simulink model "ssc_auto_ev_20b"  (R2020b)
settings: Solver=VariableStepAuto  StartTime=0.0  StopTime=200  RelTol=1e-3  AbsTol=1e-3
PreLoadFcn:
  | % Simulation parameters
  | dt = 0.01;
  | 
  | % Battery cell parameters
  | ssc_lithium_cell_1RC_ini
  | Nseries = 100;
  | Nparallel = 10;
  | 
  | % Motor parameters
  | max_torque = 220;
  | max_power = 80e3;
  | 
  | % Vehicle parameters
  | vehicle_mass = 4000;
  | wheel_radius = 0.35;
  | area = 5;
  | drag_coefficient = 0.25;
  | air_density = 1.225;
  | gravity = 9.81;
  | rolling_res_ratio = 0.015;
  | 
  | % Differential drive parameters
  | gear_ratio = 12;
  | 
  | % Simplified braking system parameters
  | force_max_pedal = 500;
  | braking_torque_to_pedal_force_ratio = -16;
  | 
  | % Vehicle controller parameters
  | hill_hold_max_speed = 0.5;
  | 
  | % Water properties for cooling circuit
  | load WaterProperties
  | 
  | % Input signals for Signal Editor block
  | load ssc_auto_ev_Inputs
values from neighbouring files (symbols this model uses):
  C1_LUT = [1913.6 4625.7 23306 10736 18036 12251 9022.9 12447 18872 40764 18721 33630 ... (21 elements, 7x3)]    [ssc_auto_ev_param.mat]
  Capacity_LUT = [28.0081 27.625 27.6392]    [ssc_auto_ev_param.mat]
  cell_Cp_heat = 810.5328    [ssc_auto_ev_param.mat]
  cell_mass = 1    [ssc_auto_ev_param.mat]
  Em_LUT = [3.4966 3.5519 3.6183 3.7066 3.9131 4.0748 4.1923 3.5057 3.566 3.6337 3.7127 3.9259 ... (21 elements, 7x3)]    [ssc_auto_ev_param.mat]
  Qe_init = 15.6845    [ssc_auto_ev_param.mat]
  R0_LUT = [0.0117 0.011 0.0114 0.0107 0.0107 0.0113 0.0116 0.0085 0.0085 0.0087 0.0082 0.0083 ... (21 elements, 7x3)]    [ssc_auto_ev_param.mat]
  R1_LUT = [0.0109 0.0069 0.0047 0.0034 0.0033 0.0033 0.0028 0.0029 0.0024 0.0026 0.0016 0.0023 ... (21 elements, 7x3)]    [ssc_auto_ev_param.mat]
  SOC_LUT = [0 0.1 0.25 0.5 0.75 0.9 1]    [ssc_auto_ev_param.mat]
  T_init = 293.15    [ssc_auto_ev_param.mat]
  Temperature_LUT = [278.15 293.15 313.15]    [ssc_auto_ev_param.mat]
undefined symbols (not defined in the file or in its folder): DiscIntNeverNeededParam, K, Lambda, tau, x0
libraries: fl_lib x656, nesl_utility x86, simulink x21, LiBatteryElements_lib x16, SignalEditorBlockLib x4, simulink_extras x4
(part 7 of 13)

== system ssc_auto_ev_20b/Step 4: Deployment Model/Vehicle and drive @100Hz ==
  Test data : Inport
  iRef : Inport  Port=2
  voltage : Inport  Port=3
  heat flow : Inport  Port=4
  heat flow1 : Inport  Port=5
  ERef2 : fl_lib/Electrical/Electrical Elements/Electrical Reference
      settings: SourceProductBaseCode=PW,SS,VE
  Motor Drive : Subsystem  Tag=PublishSubsystem  VariantControl=Variant1
  Port 1 Interface1 : Subsystem  mask(Network Coupler (Thermal Mass) Port 1 Interface){thermalMass=10*447, samplingType=physmod:simscape:couplers:SimscapeNetworkCouplersLib:VariableStepAtPorts1And2_PV, h1=dt, h2=dt*5, predictionDiscreteToContinuous=off, smoothingContinuousToDiscrete=off, predictionSlowToFast=off, smoothingFastToSlow=off, nSmooth=1, tsSmoothing=0.01, thermalConductanceNetwork=1, hRecommended=0.001, T0=T_init}
      mask prompts: thermalMass "physmod:simscape:couplers:SimscapeNetworkCouplersLib:ThermalMassJK_MP"; samplingType "physmod:simscape:couplers:SimscapeNetworkCouplersLib:SamplingType_MP"; h1 "physmod:simscape:couplers:SimscapeNetworkCouplersLib:Port1NetworkDiscreteSampleTimes_MP"; h2 "physmod:simscape:couplers:SimscapeNetworkCouplersLib:Port2NetworkDiscreteSampleTimes_MP"; predictionDiscreteToContinuous "physmod:simscape:couplers:SimscapeNetworkCouplersLib:UsePredictionWhenConnectingFixedStepToVariableStep_MP"; smoothingContinuousToDiscrete "physmod:simscape:couplers:SimscapeNetworkCouplersLib:UseSmoothingWhenConnectingVariableStepToFixedStep_MP"; predictionSlowToFast "physmod:simscape:couplers:SimscapeNetworkCouplersLib:UsePredictionWhenConnectingSlowToFastSampleTimes_MP"; smoothingFastToSlow "physmod:simscape:couplers:SimscapeNetworkCouplersLib:UseSmoothingWhenConnectingFastToSlowSampleTimes_MP"; nSmooth "physmod:simscape:couplers:SimscapeNetworkCouplersLib:NumberOfSamplesOverWhichToSmooth_MP"; tsSmoothing "physmod:simscape:couplers:SimscapeNetworkCouplersLib:SmoothingTimeConstants_MP"; thermalConductanceNetwork "physmod:simscape:couplers:SimscapeNetworkCouplersLib:ApproximateConnectedNetworkThermalConductanceWK_MP"; hRecommended "physmod:simscape:couplers:SimscapeNetworkCouplersLib:RecommendedMaxDiscreteSampleTimes_MP"; T0 "physmod:simscape:couplers:SimscapeNetworkCouplersLib:InitialTemperatureK_MP"
      mask help: physmod:simscape:couplers:SimscapeNetworkCouplersLib:NetworkCouplerThermalMassPort1Interface_MD
      mask init: same as ssc_auto_ev_20b/Step 3: Ungroup and Redraw/Port 1 Interface1
      settings: PortSchema="{\"entries\":[{\"content\":{\"sides\":[{\"content\":{\"connectorIds\":[\"LConn1\"]},\"type\":\"ConnectorPlacement.EquallySpacedRectSide\",\"uuid\":\"a6d4a9fd-b5aa-40dc-ab7e-2b646b9b57bc\"},{\"content\":{\"connectorIds\":[\"Out1\",\"In1\"],\"side\":\"RIGHT\"},\"type\":\"ConnectorPlacement.EquallySpacedRectSide\",\"uuid\":\"31bb6273-5b9b-48d0-a1a2-6fbacb979b97\"},{\"content\":{\"connectorIds\":[],\"side\":\"TOP\"},\"type\":\"ConnectorPlacement.EquallySpacedRectSide\",\"uuid\":\"0f7afab2-4481-486c-9ad0-2b42c5b091a4\"}]},\"type\":\"ConnectorPlacement.EquallySpacedConnector\",\"uuid\":\"a98e47aa-cbfd-441a-b14c-c9ea515c056e\"}],\"packageUris\":[\"http://schema.mathworks.com/mf0/Connector/R2020b\"],\"version\":\"1.0\"}"
      mask Help: web([docroot '/physmod/simscape/ref/networkcouplerthermalmass.html'])
      mask TypeOptions samplingType: physmod:simscape:couplers:SimscapeNetworkCouplersLib:VariableStepAtPorts1And2_PV | physmod:simscape:couplers:SimscapeNetworkCouplersLib:VariableStepAtPort1AndFixedStepAtPort2_PV | physmod:simscape:couplers:SimscapeNetworkCouplersLib:FixedStepBothPortsWithCommonSampleTime_PV | physmod:simscape:couplers:SimscapeNetworkCouplersLib:FixedStepBothPortsWithFasterSamplingAtPort1_PV
      mask Callback samplingType: foundation.internal.couplers.thermal.parameterVisibilitiesThermalMass(gcb)
      mask Callback predictionDiscreteToContinuous: foundation.internal.couplers.thermal.parameterVisibilitiesThermalMass(gcb)
      mask Callback smoothingContinuousToDiscrete: foundation.internal.couplers.thermal.parameterVisibilitiesThermalMass(gcb)
      mask Callback predictionSlowToFast: foundation.internal.couplers.thermal.parameterVisibilitiesThermalMass(gcb)
      mask Callback smoothingFastToSlow: foundation.internal.couplers.thermal.parameterVisibilitiesThermalMass(gcb)
      mask DialogControl Main Prompt: Main
      mask DialogControl Analysis Prompt: Analysis
      mask DialogControl connectedNetworkInfo Prompt: Connected network information
      mask DialogControl derivedValues Prompt: Derived values
      mask DialogControl updateRecommendations Prompt: Update
      mask DialogControl updateRecommendations Callback: foundation.internal.couplers.thermal.analysisThermalMass(gcb);
      mask DialogControl InitialConditions Prompt: Initial Conditions
  Port 1 Interface2 : Subsystem  mask(Network Coupler (Thermal Mass) Port 1 Interface){thermalMass=10*447, samplingType=physmod:simscape:couplers:SimscapeNetworkCouplersLib:VariableStepAtPorts1And2_PV, h1=dt, h2=dt*5, predictionDiscreteToContinuous=off, smoothingContinuousToDiscrete=off, predictionSlowToFast=off, smoothingFastToSlow=off, nSmooth=1, tsSmoothing=0.01, thermalConductanceNetwork=1, hRecommended=0.001, T0=T_init}
      mask prompts: thermalMass "physmod:simscape:couplers:SimscapeNetworkCouplersLib:ThermalMassJK_MP"; samplingType "physmod:simscape:couplers:SimscapeNetworkCouplersLib:SamplingType_MP"; h1 "physmod:simscape:couplers:SimscapeNetworkCouplersLib:Port1NetworkDiscreteSampleTimes_MP"; h2 "physmod:simscape:couplers:SimscapeNetworkCouplersLib:Port2NetworkDiscreteSampleTimes_MP"; predictionDiscreteToContinuous "physmod:simscape:couplers:SimscapeNetworkCouplersLib:UsePredictionWhenConnectingFixedStepToVariableStep_MP"; smoothingContinuousToDiscrete "physmod:simscape:couplers:SimscapeNetworkCouplersLib:UseSmoothingWhenConnectingVariableStepToFixedStep_MP"; predictionSlowToFast "physmod:simscape:couplers:SimscapeNetworkCouplersLib:UsePredictionWhenConnectingSlowToFastSampleTimes_MP"; smoothingFastToSlow "physmod:simscape:couplers:SimscapeNetworkCouplersLib:UseSmoothingWhenConnectingFastToSlowSampleTimes_MP"; nSmooth "physmod:simscape:couplers:SimscapeNetworkCouplersLib:NumberOfSamplesOverWhichToSmooth_MP"; tsSmoothing "physmod:simscape:couplers:SimscapeNetworkCouplersLib:SmoothingTimeConstants_MP"; thermalConductanceNetwork "physmod:simscape:couplers:SimscapeNetworkCouplersLib:ApproximateConnectedNetworkThermalConductanceWK_MP"; hRecommended "physmod:simscape:couplers:SimscapeNetworkCouplersLib:RecommendedMaxDiscreteSampleTimes_MP"; T0 "physmod:simscape:couplers:SimscapeNetworkCouplersLib:InitialTemperatureK_MP"
      mask help: physmod:simscape:couplers:SimscapeNetworkCouplersLib:NetworkCouplerThermalMassPort1Interface_MD
      mask init: same as ssc_auto_ev_20b/Step 3: Ungroup and Redraw/Port 1 Interface1
      settings: PortSchema="{\"entries\":[{\"content\":{\"sides\":[{\"content\":{\"connectorIds\":[\"LConn1\"]},\"type\":\"ConnectorPlacement.EquallySpacedRectSide\",\"uuid\":\"a6d4a9fd-b5aa-40dc-ab7e-2b646b9b57bc\"},{\"content\":{\"connectorIds\":[\"Out1\",\"In1\"],\"side\":\"RIGHT\"},\"type\":\"ConnectorPlacement.EquallySpacedRectSide\",\"uuid\":\"31bb6273-5b9b-48d0-a1a2-6fbacb979b97\"},{\"content\":{\"connectorIds\":[],\"side\":\"TOP\"},\"type\":\"ConnectorPlacement.EquallySpacedRectSide\",\"uuid\":\"0f7afab2-4481-486c-9ad0-2b42c5b091a4\"}]},\"type\":\"ConnectorPlacement.EquallySpacedConnector\",\"uuid\":\"a98e47aa-cbfd-441a-b14c-c9ea515c056e\"}],\"packageUris\":[\"http://schema.mathworks.com/mf0/Connector/R2020b\"],\"version\":\"1.0\"}"
      mask Help: web([docroot '/physmod/simscape/ref/networkcouplerthermalmass.html'])
      mask TypeOptions samplingType: physmod:simscape:couplers:SimscapeNetworkCouplersLib:VariableStepAtPorts1And2_PV | physmod:simscape:couplers:SimscapeNetworkCouplersLib:VariableStepAtPort1AndFixedStepAtPort2_PV | physmod:simscape:couplers:SimscapeNetworkCouplersLib:FixedStepBothPortsWithCommonSampleTime_PV | physmod:simscape:couplers:SimscapeNetworkCouplersLib:FixedStepBothPortsWithFasterSamplingAtPort1_PV
      mask Callback samplingType: foundation.internal.couplers.thermal.parameterVisibilitiesThermalMass(gcb)
      mask Callback predictionDiscreteToContinuous: foundation.internal.couplers.thermal.parameterVisibilitiesThermalMass(gcb)
      mask Callback smoothingContinuousToDiscrete: foundation.internal.couplers.thermal.parameterVisibilitiesThermalMass(gcb)
      mask Callback predictionSlowToFast: foundation.internal.couplers.thermal.parameterVisibilitiesThermalMass(gcb)
      mask Callback smoothingFastToSlow: foundation.internal.couplers.thermal.parameterVisibilitiesThermalMass(gcb)
      mask DialogControl Main Prompt: Main
      mask DialogControl Analysis Prompt: Analysis
      mask DialogControl connectedNetworkInfo Prompt: Connected network information
      mask DialogControl derivedValues Prompt: Derived values
      mask DialogControl updateRecommendations Prompt: Update
      mask DialogControl updateRecommendations Callback: foundation.internal.couplers.thermal.analysisThermalMass(gcb);
      mask DialogControl InitialConditions Prompt: Initial Conditions
  Port 1 Interface3 : Subsystem  mask(Network Coupler (Voltage-Current) Port 1 Interface){samplingType=physmod:simscape:couplers:SimscapeNetworkCouplersLib:VariableStepAtPorts1And2_PV, ts=1e-3, h1=dt, h2=dt*2, predictionDiscreteToContinuous=off, smoothingContinuousToDiscrete=off, predictionSlowToFast=off, smoothingFastToSlow=off, nSmooth=1, tsSmoothing=0.01, tsMax=1, tau=0.2, i0=0, v0=0}
      mask prompts: samplingType "physmod:simscape:couplers:SimscapeNetworkCouplersLib:SamplingType_MP"; ts "physmod:simscape:couplers:SimscapeNetworkCouplersLib:SeparatorTimeConstants_MP"; h1 "physmod:simscape:couplers:SimscapeNetworkCouplersLib:Port1NetworkDiscreteSampleTimes_MP"; h2 "physmod:simscape:couplers:SimscapeNetworkCouplersLib:Port2NetworkDiscreteSampleTimes_MP"; predictionDiscreteToContinuous "physmod:simscape:couplers:SimscapeNetworkCouplersLib:UsePredictionWhenConnectingFixedStepToVariableStep_MP"; smoothingContinuousToDiscrete "physmod:simscape:couplers:SimscapeNetworkCouplersLib:UseSmoothingWhenConnectingVariableStepToFixedStep_MP"; predictionSlowToFast "physmod:simscape:couplers:SimscapeNetworkCouplersLib:UsePredictionWhenConnectingSlowToFastSampleTimes_MP"; smoothingFastToSlow "physmod:simscape:couplers:SimscapeNetworkCouplersLib:UseSmoothingWhenConnectingFastToSlowSampleTimes_MP"; nSmooth "physmod:simscape:couplers:SimscapeNetworkCouplersLib:NumberOfSamplesOverWhichToSmooth_MP"; tsSmoothing "physmod:simscape:couplers:SimscapeNetworkCouplersLib:SmoothingTimeConstants_MP"; tsMax "physmod:simscape:couplers:SimscapeNetworkCouplersLib:CalculatedFastestTrackableTimeConstants_MP"; tau "physmod:simscape:couplers:SimscapeNetworkCouplersLib:CalculatedFilterTimeConstants_MP"; i0 "physmod:simscape:couplers:SimscapeNetworkCouplersLib:InitialCurrentA_MP"; v0 "physmod:simscape:couplers:SimscapeNetworkCouplersLib:InitialVoltageV_MP"
      mask help:
      | Port 1 interface for use when breaking two Simscape(TM) networks at an electrical connection. A first-order filter is used to break algebraic constraints between the two networks.
      |
      | Connect Port 1 to the network with the higher sample rate, or the network that is variable step if interfacing fixed step and variable step networks.
      mask init: same as ssc_auto_ev_20b/Step 3: Ungroup and Redraw/Port 1 Interface3
      settings: PortSchema="{\"entries\":[{\"content\":{\"sides\":[{\"content\":{\"connectorIds\":[\"LConn1\"]},\"type\":\"ConnectorPlacement.EquallySpacedRectSide\",\"uuid\":\"a6d4a9fd-b5aa-40dc-ab7e-2b646b9b57bc\"},{\"content\":{\"connectorIds\":[\"Out1\",\"In1\"],\"side\":\"RIGHT\"},\"type\":\"ConnectorPlacement.EquallySpacedRectSide\",\"uuid\":\"31bb6273-5b9b-48d0-a1a2-6fbacb979b97\"},{\"content\":{\"connectorIds\":[],\"side\":\"TOP\"},\"type\":\"ConnectorPlacement.EquallySpacedRectSide\",\"uuid\":\"0f7afab2-4481-486c-9ad0-2b42c5b091a4\"}]},\"type\":\"ConnectorPlacement.EquallySpacedConnector\",\"uuid\":\"a98e47aa-cbfd-441a-b14c-c9ea515c056e\"}],\"packageUris\":[\"http://schema.mathworks.com/mf0/Connector/R2020b\"],\"version\":\"1.0\"}"
      mask Help: web([docroot '/physmod/simscape/ref/networkcouplervoltagecurrent.html'])
      mask TypeOptions samplingType: physmod:simscape:couplers:SimscapeNetworkCouplersLib:VariableStepAtPorts1And2_PV | physmod:simscape:couplers:SimscapeNetworkCouplersLib:VariableStepAtPort1AndFixedStepAtPort2_PV | physmod:simscape:couplers:SimscapeNetworkCouplersLib:FixedStepBothPortsWithCommonSampleTime_PV | physmod:simscape:couplers:SimscapeNetworkCouplersLib:FixedStepBothPortsWithFasterSamplingAtPort1_PV
      mask Callback samplingType: foundation.internal.couplers.electrical.parameterVisibilitiesSources(gcb)
      mask Callback predictionDiscreteToContinuous: foundation.internal.couplers.electrical.parameterVisibilitiesSources(gcb)
      mask Callback smoothingContinuousToDiscrete: foundation.internal.couplers.electrical.parameterVisibilitiesSources(gcb)
      mask Callback predictionSlowToFast: foundation.internal.couplers.electrical.parameterVisibilitiesSources(gcb)
      mask Callback smoothingFastToSlow: foundation.internal.couplers.electrical.parameterVisibilitiesSources(gcb)
      mask DialogControl Main Prompt: Main
      mask DialogControl Analysis Prompt: Analysis
      mask DialogControl updateRecommendations Prompt: Update
      mask DialogControl updateRecommendations Callback: foundation.internal.couplers.electrical.analysisSources(gcb);
      mask DialogControl InitialConditions Prompt: Initial Conditions
  Solver Configuration1 : nesl_utility/Solver Configuration  PhysicalDomain=network_engine_domain  SubClassName=solver  LeftPortType=input  RightPortType=generic  Tones=[]  Harmonics=[]  SimulateNoise=off  Profile=off  UseLocalSampling=off  EnableSwitchedLinearOptims=on  FrequencyDomain=off  UseCCode=off  RelTol=0.001  AbsTol=1e-06  MinStep=1e-09  ToWorkspace=off  RevertToSquareIcSolve=off  NumHomotopyIterations=100  PhasorMode=off  PhasorModeNumHarmonics=1  DoDC=off  ResidualTolerance=1e-9  UseLocalSolver=on  LocalSolverChoice=NE_BACKWARD_EULER_ADVANCER  LocalSolverSampleTime=dt  DoFixedCost=on  MaxNonlinIter=3  MaxModeIter=2  ComputeImpulses=off  ImpulseIterations=2  LinearAlgebra=auto  EquationFormulation=NE_TIME_EF  DelaysMemoryBudget=1024  AutomaticFiltering=on  FilteringTimeConstant=0.001  PartitionStorageMethod=AS_NEEDED  PartitionMemoryBudget=1024  PartitionMethod=FAST
      settings: AttributesFormatString=Local Solver: %<UseLocalSolver>  SourceProductBaseCode=SS,PW,VE
  Vehicle Dynamics : Subsystem
  w : Outport
  current : Outport  Port=2
  temperature : Outport  Port=3
  temperature1 : Outport  Port=4
  wires:
  voltage/1 -> Port 1 Interface3/1(voltage)
  heat flow/1 -> Port 1 Interface2/1(heat flow)
  Motor Drive/1(w) -> w/1
  Test data/1 -> Vehicle Dynamics/1(Test data)
  heat flow1/1 -> Port 1 Interface1/1(heat flow)
  Port 1 Interface1/1(temperature) -> temperature1/1
  Port 1 Interface2/1(temperature) -> temperature/1
  iRef/1 -> Motor Drive/1(iRef)
  Port 1 Interface3/1(current) -> current/1
  connections:
  ERef2/LConn1 -- Motor Drive/LConn2
  Solver Configuration1/RConn1 -- Vehicle Dynamics/LConn1 -- Motor Drive/RConn1
  Motor Drive/LConn1 -- Port 1 Interface3/LConn1
  Motor Drive/LConn3 -- Port 1 Interface2/LConn1
  Motor Drive/LConn4 -- Port 1 Interface1/LConn1

== system ssc_auto_ev_20b/Vehicle Dynamics/Brake Torque ==
  Pedal : Inport
  Force for max pedal deflection : Gain  Gain=force_max_pedal
  Ideal Torque Source : fl_lib/Mechanical/Mechanical Sources/Ideal Torque Source
      settings: SourceProductBaseCode=PW,SS,VE
  MRRef : fl_lib/Mechanical/Rotational Elements/Mechanical Rotational Reference
      settings: SourceProductBaseCode=PW,SS,VE
  Motion Sensor : fl_lib/Mechanical/Mechanical Sensors/Ideal Rotational Motion Sensor  wrap_angle=simscape.enum.onoff.off  offset=0 rad
      settings: SourceProductBaseCode=PW,SS,VE
  PS Product : fl_lib/Physical Signals/Functions/PS Product
      settings: SourceProductBaseCode=PW,SS,VE
  Simulink-PS Converter1 : nesl_utility/Simulink-PS Converter  PhysicalDomain=network_engine_domain  SubClassName=ps_input  LeftPortType=input  RightPortType=output  PseudoPeriodic=off  Frequencies=[]  NoiseDistribution=none  NoiseParameters=[]  Unit=N*m  AffineConversion=off  FilteringAndDerivatives=zero  SimscapeFilterOrder=1  InputFilterTimeConstant=0.001  UdotUserProvided=1
      settings: SourceProductBaseCode=SS,PW,VE
  Smooth Sign : Subsystem
  Torque per unit brake pedal force : Gain  Gain=braking_torque_to_pedal_force_ratio
  R : PMIOPort  Side=Right
  wires:
  Force for max pedal deflection/1 -> Torque per unit brake pedal force/1
  Pedal/1 -> Force for max pedal deflection/1
  Torque per unit brake pedal force/1 -> Simulink-PS Converter1/1
  connections:
  Smooth Sign/LConn1 -- Motion Sensor/RConn2
  PS Product/LConn2 -- Simulink-PS Converter1/RConn1
  PS Product/RConn1 -- Ideal Torque Source/RConn1
  R/RConn1 -- Motion Sensor/LConn1 -- Ideal Torque Source/LConn1
  Ideal Torque Source/RConn2 -- MRRef/LConn1 -- Motion Sensor/RConn1
  Smooth Sign/RConn1 -- PS Product/LConn1

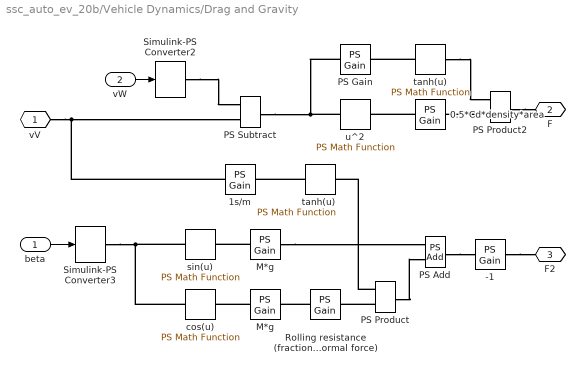
== system ssc_auto_ev_20b/Vehicle Dynamics/Drag and Gravity ==
  beta : Inport
  vW : Inport  Port=2
  " M*g " : fl_lib/Physical Signals/Functions/PS Gain  gain=vehicle_mass*gravity kg*m/s^2
      settings: SourceProductBaseCode=PW,SS,VE
  " tanh(u) " : fl_lib/Physical Signals/Functions/PS Math Function  fcn_choice=foundation.enum.math_function.tanh
      settings: SourceProductBaseCode=PW,SS,VE
  -1 : fl_lib/Physical Signals/Functions/PS Gain  gain=-1
      settings: SourceProductBaseCode=PW,SS,VE
  0.5*Cd*density*area : fl_lib/Physical Signals/Functions/PS Gain  gain=0.5*drag_coefficient*air_density*area kg/m^3*m^2
      settings: SourceProductBaseCode=PW,SS,VE
  1s/m : fl_lib/Physical Signals/Functions/PS Gain  gain=1 1/(m/s)
      settings: SourceProductBaseCode=PW,SS,VE
  M*g : fl_lib/Physical Signals/Functions/PS Gain  gain=vehicle_mass*gravity kg*m/s^2
      settings: SourceProductBaseCode=PW,SS,VE
  PS Add : fl_lib/Physical Signals/Functions/PS Add
      settings: SourceProductBaseCode=PW,SS,VE
  PS Gain : fl_lib/Physical Signals/Functions/PS Gain  gain=1 1/(m/s)
      settings: SourceProductBaseCode=PW,SS,VE
  PS Product : fl_lib/Physical Signals/Functions/PS Product
      settings: SourceProductBaseCode=PW,SS,VE
  PS Product2 : fl_lib/Physical Signals/Functions/PS Product
      settings: SourceProductBaseCode=PW,SS,VE
  PS Subtract : fl_lib/Physical Signals/Functions/PS Subtract
      settings: SourceProductBaseCode=PW,SS,VE
  Rolling resistance (fraction of normal force) : fl_lib/Physical Signals/Functions/PS Gain  gain=rolling_res_ratio
      settings: SourceProductBaseCode=PW,SS,VE
  Simulink-PS Converter2 : nesl_utility/Simulink-PS Converter  PhysicalDomain=network_engine_domain  SubClassName=ps_input  LeftPortType=input  RightPortType=output  PseudoPeriodic=off  Frequencies=[]  NoiseDistribution=none  NoiseParameters=[]  Unit=m/s  AffineConversion=off  FilteringAndDerivatives=zero  SimscapeFilterOrder=1  InputFilterTimeConstant=0.001  UdotUserProvided=1
      settings: SourceProductBaseCode=SS,PW,VE
  Simulink-PS Converter3 : nesl_utility/Simulink-PS Converter  PhysicalDomain=network_engine_domain  SubClassName=ps_input  LeftPortType=input  RightPortType=output  PseudoPeriodic=off  Frequencies=[]  NoiseDistribution=none  NoiseParameters=[]  Unit=deg  AffineConversion=off  FilteringAndDerivatives=zero  SimscapeFilterOrder=1  InputFilterTimeConstant=0.001  UdotUserProvided=1
      settings: SourceProductBaseCode=SS,PW,VE
  cos(u) : fl_lib/Physical Signals/Functions/PS Math Function  fcn_choice=foundation.enum.math_function.cos
      settings: SourceProductBaseCode=PW,SS,VE
  sin(u) : fl_lib/Physical Signals/Functions/PS Math Function  fcn_choice=foundation.enum.math_function.sin
      settings: SourceProductBaseCode=PW,SS,VE
  tanh(u) : fl_lib/Physical Signals/Functions/PS Math Function  fcn_choice=foundation.enum.math_function.tanh
      settings: SourceProductBaseCode=PW,SS,VE
  u^2 : fl_lib/Physical Signals/Functions/PS Math Function  fcn_choice=foundation.enum.math_function.square
      settings: SourceProductBaseCode=PW,SS,VE
  vV : PMIOPort  Side=Left
  F : PMIOPort  Port=2  Side=Left
  F2 : PMIOPort  Port=3  Side=Left
  wires:
  vW/1 -> Simulink-PS Converter2/1
  beta/1 -> Simulink-PS Converter3/1
  connections:
  vV/RConn1 -- 1s/m/LConn1 -- PS Subtract/LConn1
  Simulink-PS Converter2/RConn1 -- PS Subtract/LConn2
  PS Product2/RConn1 -- F/RConn1
  PS Product/LConn2 -- Rolling resistance (fraction of normal force)/RConn1
  PS Product/RConn1 -- PS Add/LConn2
  PS Add/RConn1 -- -1/LConn1
  -1/RConn1 -- F2/RConn1
  PS Product/LConn1 -- tanh(u)/RConn1
  tanh(u)/LConn1 -- 1s/m/RConn1
  PS Gain/LConn1 -- PS Subtract/RConn1 -- u^2/LConn1
  " tanh(u) "/RConn1 -- PS Product2/LConn1
  0.5*Cd*density*area/LConn1 -- u^2/RConn1
  " tanh(u) "/LConn1 -- PS Gain/RConn1
  PS Product2/LConn2 -- 0.5*Cd*density*area/RConn1
  cos(u)/LConn1 -- Simulink-PS Converter3/RConn1 -- sin(u)/LConn1
  M*g/RConn1 -- PS Add/LConn1
  Rolling resistance (fraction of normal force)/LConn1 -- " M*g "/RConn1
  M*g/LConn1 -- sin(u)/RConn1
  " M*g "/LConn1 -- cos(u)/RConn1

== system ssc_auto_ev_20b/Vehicle Dynamics/Sensing Speed ==
  MTRef : fl_lib/Mechanical/Translational Elements/Mechanical Translational Reference
      settings: SourceProductBaseCode=PW,SS,VE
  Motion Sensor : fl_lib/Mechanical/Mechanical Sensors/Ideal Translational Motion Sensor  offset=0 m
      settings: SourceProductBaseCode=PW,SS,VE
  R : PMIOPort  Side=Left
  w : PMIOPort  Port=2  Side=Right
  connections:
  Motion Sensor/RConn2 -- w/RConn1
  MTRef/LConn1 -- Motion Sensor/RConn1
  R/RConn1 -- Motion Sensor/LConn1

== system ssc_auto_ev_20b/Vehicle Control/Cruise Control ==
  Enable : Inport
  Disable : Inport  Port=2
  wMeas : Inport  Port=3
  Brake sw : Inport  Port=4
  Capture speed : Subsystem  TreatAsAtomicUnit=on
  Data Type Conversion1 : DataTypeConversion  OutDataTypeStr=boolean
  J-K Flip-Flop : simulink_extras/Flip Flops/J-K Flip-Flop  initial_condition=0
  Logical Operator : Logic  Operator=OR  AllPortsSameDT=off  OutDataTypeStr=boolean
  Pulse Generator : DiscretePulseGenerator  Period=10  PulseWidth=5  SampleTime=0.01
  Speed Controller : Subsystem  mask(P+I motor speed controller){Kp=100, Ki=100, trqMax=max_torque, ts=dt}
      mask prompts: Kp "Proportional gain (Nm/(rad/s))"; Ki "Integral gain (Nm/rad)"; trqMax "Maximum torque demand"; ts "Sample time"
      mask help: Inputs wRef and wMeas are the demanded rotor speed and measured rotor speed in rad/s. The controller output is a torque demand in Nm.
  Terminator : Terminator
  trqRef : Outport  VectorParamsAs1DForOutWhenUnconnected=off
  Enabled : Outport  Port=2  VectorParamsAs1DForOutWhenUnconnected=off
  wires:
  Capture speed/1(Out1) -> Speed Controller/1(wRef)
  J-K Flip-Flop/2 -> Terminator/1
  Data Type Conversion1/1 -> J-K Flip-Flop/1
  J-K Flip-Flop/1 -> Capture speed/Trigger, Enabled/1
  Logical Operator/1 -> J-K Flip-Flop/3
  wMeas/1 -> Speed Controller/2(wMeas), Capture speed/1(In1)
  Brake sw/1 -> Logical Operator/2
  Speed Controller/1(trqRef) -> trqRef/1
  Disable/1 -> Logical Operator/1
  Pulse Generator/1 -> J-K Flip-Flop/2
  Enable/1 -> Data Type Conversion1/1

== system ssc_auto_ev_20b/Vehicle Control/Feedforward term for regenerative braking on downhill ==
  Inclin. : Inport
  " M " : Gain  Gain=vehicle_mass
  1/ratio : Gain  Gain=1/gear_ratio
  Two motors : Gain  Gain=0.5
  Wheel radius : Gain  Gain=wheel_radius
  "[-inf,0]" : Saturate  UpperLimit=0  LowerLimit=-inf
  Feedfwd trq : Outport  VectorParamsAs1DForOutWhenUnconnected=off
  wires:
  Wheel radius/1 -> 1/ratio/1  "Wheel torque"
  " M "/1 -> Wheel radius/1
  Inclin./1 -> "[-inf,0]"/1
  "[-inf,0]"/1 -> " M "/1
  1/ratio/1 -> Two motors/1  "Motor torque"
  Two motors/1 -> Feedfwd trq/1

== system ssc_auto_ev_20b/Vehicle Control/Max Power ==
  Vspd : Inport
  Abs : Abs
  Constant : Constant
  Math Function : Math  Operator=reciprocal  SignedPower=on  SaturateOnIntegerOverflow=on
  Prevent divide by zero : Switch  Criteria=u2 > Threshold  Threshold=1
  max_power : Gain  Gain=max_power
  Max Power : Outport  VectorParamsAs1DForOutWhenUnconnected=off
  wires:
  Vspd/1 -> Abs/1
  max_power/1 -> Max Power/1
  Math Function/1 -> max_power/1
  Abs/1 -> Prevent divide by zero/1, Prevent divide by zero/2
  Constant/1 -> Prevent divide by zero/3
  Prevent divide by zero/1 -> Math Function/1

== system ssc_auto_ev_20b/Vehicle Control/Torque Demand Management ==
  Brake : Inport
  Throttle : Inport  Port=2
  wMeas : Inport  Port=3
  FFbrake : Inport  Port=4
  1/ratio : Gain  Gain=1/gear_ratio
  Disable braking at low and negative speeds : Lookup_n-D  NumberOfTableDimensions=1  BreakpointsForDimension1=[-100 -1 0 5 10 100]  Table=[0 0 0 0 1 1]  InternalRulePriority=Speed  RndMeth=Simplest  InputSameDT=on
  Disable braking at low and negative speeds1 : Lookup_n-D  NumberOfTableDimensions=1  BreakpointsForDimension1=[-100 -1 0 5 10 100]  Table=[0 0 0 0 1 1]  InternalRulePriority=Speed  RndMeth=Simplest  InputSameDT=on
  Force for max pedal deflection : Gain  Gain=force_max_pedal
  Max torque demand : Gain  Gain=max_torque
  Motor torque limits2 : Saturate  UpperLimit=max_torque  LowerLimit=-max_torque
  Product : Product
  Product1 : Product
  Sum : Sum  Inputs=|++
  Sum1 : Sum  Inputs=|++
  Torque per unit brake pedal force : Gain  Gain=braking_torque_to_pedal_force_ratio
  Two motors : Gain  Gain=1/2
  wMeas1 : InportShadow  Port=3
  Dem trq : Outport  VectorParamsAs1DForOutWhenUnconnected=off
  wires:
  Two motors/1 -> Product/1
  Product/1 -> Sum/2
  wMeas/1 -> Disable braking at low and negative speeds/1
  Force for max pedal deflection/1 -> Torque per unit brake pedal force/1
  1/ratio/1 -> Two motors/1
  Torque per unit brake pedal force/1 -> 1/ratio/1
  Throttle/1 -> Max torque demand/1
  Brake/1 -> Force for max pedal deflection/1
  Max torque demand/1 -> Sum/1
  Sum/1 -> Sum1/1
  Disable braking at low and negative speeds/1 -> Product/2
  FFbrake/1 -> Product1/1
  Disable braking at low and negative speeds1/1 -> Product1/2
  wMeas1/1 -> Disable braking at low and negative speeds1/1
  Product1/1 -> Sum1/2
  Sum1/1 -> Motor torque limits2/1
  Motor torque limits2/1 -> Dem trq/1

== system ssc_auto_ev_20b/Battery/Electric and Thermal Model/Thermal Model ==
  Heat Flow Source : fl_lib/Thermal/Thermal Sources/Controlled Heat Flow Rate Source
      settings: SourceProductBaseCode=PW,SS,VE
  Ideal Temperature Sensor : fl_lib/Thermal/Thermal Sensors/Temperature Sensor
      settings: SourceProductBaseCode=PW,SS,VE
  ThRef1 : fl_lib/Thermal/Thermal Elements/Thermal Reference
      settings: SourceProductBaseCode=PW,SS,VE
  ThRef2 : fl_lib/Thermal/Thermal Elements/Thermal Reference
      settings: SourceProductBaseCode=PW,SS,VE
  PlossTotal : PMIOPort  Tag=PMCPort  Side=Left
  T : PMIOPort  Tag=PMCPort  Port=2  Side=Right
  H : PMIOPort  Tag=PMCPort  Port=3  Side=Left
  connections:
  Heat Flow Source/RConn1 -- PlossTotal/RConn1
  Heat Flow Source/LConn1 -- H/RConn1 -- Ideal Temperature Sensor/LConn1
  ThRef1/LConn1 -- Heat Flow Source/RConn2
  Ideal Temperature Sensor/RConn2 -- T/RConn1
  ThRef2/LConn1 -- Ideal Temperature Sensor/RConn1

== system ssc_auto_ev_20b/Cooling System/ Heat Exchanger Characteristic/Characteristic ==
  PS Product : fl_lib/Physical Signals/Functions/PS Product
      settings: SourceProductBaseCode=PW,SS,VE
  PS Subtract : fl_lib/Physical Signals/Functions/PS Subtract
      settings: SourceProductBaseCode=PW,SS,VE
  Specific dissipation (J/s/K) per unit mass flow rate : fl_lib/Physical Signals/Functions/PS Gain  gain=100 J/s/(kg/s)/K
      settings: SourceProductBaseCode=PW,SS,VE
  M : PMIOPort  Side=Right
  T in : PMIOPort  Port=2  Side=Right
  T Env : PMIOPort  Port=3  Side=Right
  Q : PMIOPort  Port=4  Side=Left
  connections:
  PS Product/LConn2 -- Specific dissipation (J/s/K) per unit mass flow rate/RConn1
  Specific dissipation (J/s/K) per unit mass flow rate/LConn1 -- M/RConn1
  PS Subtract/LConn2 -- T in/RConn1
  PS Subtract/RConn1 -- PS Product/LConn1
  PS Product/RConn1 -- Q/RConn1
  PS Subtract/LConn1 -- T Env/RConn1

== system ssc_auto_ev_20b/Cooling System/Heat Exchanger Characteristic/Characteristic ==
  PS Product1 : fl_lib/Physical Signals/Functions/PS Product
      settings: SourceProductBaseCode=PW,SS,VE
  PS Subtract : fl_lib/Physical Signals/Functions/PS Subtract
      settings: SourceProductBaseCode=PW,SS,VE
  Specific dissipation : fl_lib/Physical Signals/Lookup Tables/PS Lookup Table (1D)  x="[0 0.2 0.4  0.7  1 1.2  1.4  2.5 ] kg/s"  f=10000 * [0 0.5 0.75 0.92 1 1.02 1.03 1.04] J/s/K  interp_method=simscape.enum.interpolation.linear  extrap_method=simscape.enum.extrapolation.linear
      settings: SourceProductBaseCode=PW,SS,VE
  Mass Flow : PMIOPort  Side=Left
  Temp Inlet : PMIOPort  Port=2  Side=Left
  Temp Motor : PMIOPort  Port=3  Side=Left
  Q : PMIOPort  Port=4  Side=Right
  connections:
  Specific dissipation/LConn1 -- Mass Flow/RConn1
  Q/RConn1 -- PS Product1/RConn1
  PS Subtract/LConn2 -- Temp Inlet/RConn1
  PS Subtract/LConn1 -- Temp Motor/RConn1
  PS Product1/LConn2 -- Specific dissipation/RConn1
  PS Product1/LConn1 -- PS Subtract/RConn1

== system ssc_auto_ev_20b/Step 2: Multirate Model/Battery/Electric and Thermal Model ==
  note: Equivalent Circuit Model for Single Battery Cell
  C1 : LiBatteryElements_lib/C_table  C_Table=C1_LUT*Nparallel F  SOC_Table=SOC_LUT  Temp_Table=Temperature_LUT K  v0=0 V
      settings: SourceProductBaseCode=SS  InternalSimscapePortConfiguration="{\"Bottom\":[],\"Left\":[{\"id\":\"p\",\"label\":\"+\",\"type\":\"foundation.electrical.electrical\"},{\"id\":\"T\",\"label\":\"T\",\"type\":\"input\"},{\"id\":\"SOC\",\"label\":\"SOC\",\"type\":\"input\"}],\"Right\":[{\"id\":\"n\",\"label\":\"-\",\"type\":\"foundation.electrical.electrical\"}],\"Top\":[]}"
  Em_table : LiBatteryElements_lib/Em_table  C_Table=Capacity_LUT*Nparallel hr*A  Em_Table=Em_LUT V  SOC_Table=SOC_LUT  Temp_Table=Temperature_LUT K  Qinit=Qe_init*Nparallel hr*A
      settings: SourceProductBaseCode=SS  InternalSimscapePortConfiguration="{\"Bottom\":[],\"Left\":[{\"id\":\"p\",\"label\":\"+\",\"type\":\"foundation.electrical.electrical\"},{\"id\":\"C\",\"label\":\"C\",\"type\":\"output\"},{\"id\":\"SOC\",\"label\":\"SOC\",\"type\":\"output\"}],\"Right\":[{\"id\":\"n\",\"label\":\"-\",\"type\":\"foundation.electrical.electrical\"},{\"id\":\"T\",\"label\":\"T\",\"type\":\"input\"}],\"Top\":[]}"
  NumCells : fl_lib/Physical Signals/Functions/PS Gain  gain=Nseries
      settings: SourceProductBaseCode=PW,SS,VE
  PS Add : fl_lib/Physical Signals/Functions/PS Add
      settings: SourceProductBaseCode=PW,SS,VE
  R0 : LiBatteryElements_lib/R_table  R_Table=R0_LUT/Nparallel Ohm  SOC_Table=SOC_LUT  Temp_Table=Temperature_LUT K
      settings: SourceProductBaseCode=SS  InternalSimscapePortConfiguration="{\"Bottom\":[],\"Left\":[{\"id\":\"p\",\"label\":\"+\",\"type\":\"foundation.electrical.electrical\"},{\"id\":\"T\",\"label\":\"T\",\"type\":\"input\"},{\"id\":\"SOC\",\"label\":\"SOC\",\"type\":\"input\"}],\"Right\":[{\"id\":\"n\",\"label\":\"-\",\"type\":\"foundation.electrical.electrical\"},{\"id\":\"pow\",\"label\":\"POW\",\"type\":\"output\"}],\"Top\":[]}"
  R1 : LiBatteryElements_lib/R_table  R_Table=R1_LUT/Nparallel Ohm  SOC_Table=SOC_LUT  Temp_Table=Temperature_LUT K
      settings: SourceProductBaseCode=SS  InternalSimscapePortConfiguration="{\"Bottom\":[],\"Left\":[{\"id\":\"p\",\"label\":\"+\",\"type\":\"foundation.electrical.electrical\"},{\"id\":\"T\",\"label\":\"T\",\"type\":\"input\"},{\"id\":\"SOC\",\"label\":\"SOC\",\"type\":\"input\"}],\"Right\":[{\"id\":\"n\",\"label\":\"-\",\"type\":\"foundation.electrical.electrical\"},{\"id\":\"pow\",\"label\":\"POW\",\"type\":\"output\"}],\"Top\":[]}"
  Thermal Model : Subsystem
  + : PMIOPort  Side=Right
  - : PMIOPort  Port=2  Side=Right
  H : PMIOPort  Tag=PMCPort  Port=3  Side=Left
  connections:
  H/RConn1 -- Thermal Model/LConn2
  NumCells/RConn1 -- Thermal Model/LConn1
  R1/LConn3 -- C1/LConn3 -- Em_table/LConn3 -- R0/LConn3
  Em_table/RConn1 -- -/RConn1
  R0/LConn1 -- R1/RConn1 -- C1/RConn1
  PS Add/LConn1 -- R0/RConn2
  PS Add/LConn2 -- R1/RConn2
  C1/LConn1 -- R1/LConn1 -- Em_table/LConn1
  R1/LConn2 -- Thermal Model/RConn1 -- Em_table/RConn2 -- R0/LConn2 -- C1/LConn2
  +/RConn1 -- R0/RConn1
  PS Add/RConn1 -- NumCells/LConn1

== system ssc_auto_ev_20b/Step 2: Multirate Model/Battery Thermal Mass/Port 1 Interface ==
  heat flow : Inport
  Controlled Temperature Source : fl_lib/Thermal/Thermal Sources/Controlled Temperature Source
      settings: SourceProductBaseCode=PW,SS,VE
  Heat Flow Rate Sensor : fl_lib/Thermal/Thermal Sensors/Heat Flow Rate Sensor
      settings: SourceProductBaseCode=PW,SS,VE
  Interface : Subsystem  Variant=on  VariantControlMode=label  VariantControl=Variant1  LabelModeActiveChoice=Discrete
      settings: PortSchema="{\"entries\":[{\"content\":{\"sides\":[{\"content\":{\"connectorIds\":[\"In1\",\"Out2\"]},\"type\":\"ConnectorPlacement.EquallySpacedRectSide\",\"uuid\":\"aa56821c-7799-44e3-b228-553c5b43a68d\"},{\"content\":{\"connectorIds\":[\"In2\",\"Out1\"],\"side\":\"RIGHT\"},\"type\":\"ConnectorPlacement.EquallySpacedRectSide\",\"uuid\":\"8658dee5-55e2-4f33-bdec-e6600ce27fc1\"},{\"content\":{\"connectorIds\":[],\"side\":\"TOP\"},\"type\":\"ConnectorPlacement.EquallySpacedRectSide\",\"uuid\":\"2effe9c6-8e61-4f0c-a39b-329d9ffc707d\"}]},\"type\":\"ConnectorPlacement.EquallySpacedConnector\",\"uuid\":\"c8fc8444-dfc7-49a5-9550-b957635f7d8f\"}],\"packageUris\":[\"http://schema.mathworks.com/mf0/Connector/R2020b\"],\"version\":\"1.0\"}"
  T1 : nesl_utility/Simulink-PS Converter  PhysicalDomain=network_engine_domain  SubClassName=ps_input  LeftPortType=input  RightPortType=output  PseudoPeriodic=off  Frequencies=[]  NoiseDistribution=none  NoiseParameters=[]  Unit=K  AffineConversion=off  FilteringAndDerivatives=provide  SimscapeFilterOrder=1  InputFilterTimeConstant=0.001  UdotUserProvided=0
      settings: SourceProductBaseCode=SS,PW,VE
  Thermal Reference : fl_lib/Thermal/Thermal Elements/Thermal Reference
      settings: SourceProductBaseCode=PW,SS,VE
  q1 : nesl_utility/PS-Simulink Converter  PhysicalDomain=network_engine_domain  SubClassName=ps_output  LeftPortType=input  RightPortType=output  PseudoPeriodic=off  Frequencies=[]  Unit=W  AffineConversion=off
      settings: SourceProductBaseCode=SS,PW,VE
  1 : PMIOPort  Side=Left
  temperature : Outport
  wires:
  Interface/2(across1) -> T1/1
  heat flow/1 -> Interface/2(through2)
  q1/1 -> Interface/1(through1)
  Interface/1(across2) -> temperature/1
  connections:
  Controlled Temperature Source/RConn1 -- T1/RConn1
  Thermal Reference/LConn1 -- Controlled Temperature Source/RConn2
  q1/LConn1 -- Heat Flow Rate Sensor/RConn1
  Heat Flow Rate Sensor/LConn1 -- 1/RConn1
  Heat Flow Rate Sensor/RConn2 -- Controlled Temperature Source/LConn1

== system ssc_auto_ev_20b/Step 2: Multirate Model/Battery Thermal Mass/Port 2 Interface ==
  temperature : Inport
  Controlled Temperature Source : fl_lib/Thermal/Thermal Sources/Controlled Temperature Source
      settings: SourceProductBaseCode=PW,SS,VE
  Heat Flow Rate Sensor : fl_lib/Thermal/Thermal Sensors/Heat Flow Rate Sensor
      settings: SourceProductBaseCode=PW,SS,VE
  T2 : nesl_utility/Simulink-PS Converter  PhysicalDomain=network_engine_domain  SubClassName=ps_input  LeftPortType=input  RightPortType=output  PseudoPeriodic=off  Frequencies=[]  NoiseDistribution=none  NoiseParameters=[]  Unit=K  AffineConversion=off  FilteringAndDerivatives=provide  SimscapeFilterOrder=1  InputFilterTimeConstant=0.001  UdotUserProvided=0
      settings: SourceProductBaseCode=SS,PW,VE
  Thermal Reference : fl_lib/Thermal/Thermal Elements/Thermal Reference
      settings: SourceProductBaseCode=PW,SS,VE
  q2 : nesl_utility/PS-Simulink Converter  PhysicalDomain=network_engine_domain  SubClassName=ps_output  LeftPortType=input  RightPortType=output  PseudoPeriodic=off  Frequencies=[]  Unit=W  AffineConversion=off
      settings: SourceProductBaseCode=SS,PW,VE
  2 : PMIOPort  Side=Right
  heat flow : Outport
  wires:
  temperature/1 -> T2/1
  q2/1 -> heat flow/1
  connections:
  q2/LConn1 -- Heat Flow Rate Sensor/RConn1
  T2/RConn1 -- Controlled Temperature Source/RConn1
  Heat Flow Rate Sensor/LConn1 -- 2/RConn1
  Thermal Reference/LConn1 -- Controlled Temperature Source/RConn2
  Heat Flow Rate Sensor/RConn2 -- Controlled Temperature Source/LConn1

== system ssc_auto_ev_20b/Step 2: Multirate Model/Cooling System/ Heat Exchanger Characteristic ==
  Characteristic : Subsystem
  Heat Flow Source : fl_lib/Thermal/Thermal Sources/Controlled Heat Flow Rate Source
      settings: SourceProductBaseCode=PW,SS,VE
  Mass Flow Rate & Thermal Flux Sensor (TL) : fl_lib/Thermal Liquid/Sensors/Mass & Energy Flow Rate Sensor (TL)
      settings: SourceProductBaseCode=PW,SS,VE  InternalSimscapePortConfiguration="{\"Bottom\":[],\"Left\":[{\"id\":\"A\",\"label\":\"A\",\"type\":\"foundation.thermal_liquid.thermal_liquid\"}],\"Right\":[{\"id\":\"B\",\"label\":\"B\",\"type\":\"foundation.thermal_liquid.thermal_liquid\"},{\"id\":\"M\",\"label\":\"M\",\"type\":\"output\"},{\"id\":\"PHI\",\"label\":\"Phi\",\"type\":\"output\"}],\"Top\":[]}"
  Temperature Sensor : fl_lib/Thermal/Thermal Sensors/Temperature Sensor
      settings: SourceProductBaseCode=PW,SS,VE
  ThRef : fl_lib/Thermal/Thermal Elements/Thermal Reference
      settings: SourceProductBaseCode=PW,SS,VE
  Henv : PMIOPort  Side=Right
  Hp : PMIOPort  Port=2  Side=Left
  B : PMIOPort  Port=3  Side=Right
  Phi : PMIOPort  Port=4  Side=Right
  A : PMIOPort  Port=5  Side=Left
  T in : PMIOPort  Port=6  Side=Left
  connections:
  Characteristic/LConn1 -- Heat Flow Source/RConn1
  Temperature Sensor/RConn2 -- Characteristic/RConn3
  T in/RConn1 -- Characteristic/RConn2
  Mass Flow Rate & Thermal Flux Sensor (TL)/RConn2 -- Characteristic/RConn1
  Mass Flow Rate & Thermal Flux Sensor (TL)/RConn3 -- Phi/RConn1
  Mass Flow Rate & Thermal Flux Sensor (TL)/RConn1 -- B/RConn1
  Heat Flow Source/LConn1 -- Hp/RConn1
  ThRef/LConn1 -- Temperature Sensor/RConn1
  Heat Flow Source/RConn2 -- Henv/RConn1 -- Temperature Sensor/LConn1
  A/RConn1 -- Mass Flow Rate & Thermal Flux Sensor (TL)/LConn1

== system ssc_auto_ev_20b/Step 2: Multirate Model/Cooling System/Expansion Tank ==
  Air Stiffness : fl_lib/Mechanical/Translational Elements/Translational Spring  spr_rate=1e3 N/m  v_specify=off  v_priority=High  v=0 m/s  v_nominal_specify=off  v_nominal_unit=m/s  v_nominal_value=1  f_specify=on  f_priority=Low  f=0 N  f_nominal_specify=off  f_nominal_unit=N  f_nominal_value=1  x_specify=off  x_priority=High  x=0 m  x_nominal_specify=off  x_nominal_unit=m  x_nominal_value=1
      settings: SourceProductBaseCode=PW,SS,VE
  Expansion Tank : fl_lib/Thermal Liquid/Elements/Translational Mechanical Converter (TL)  mech_orientation=1  interface_area=pi*50^2 mm^2  x0=200 mm  dead_volume=0.001 m^3  environment_spec=1  environment_pressure=0.101325 MPa  dynamic_compressibility=0  p0=1 atm  T0=20 degC
      settings: SourceProductBaseCode=PW,SS,VE  InternalSimscapePortConfiguration="{\"Bottom\":[],\"Left\":[{\"id\":\"A\",\"label\":\"A\",\"type\":\"foundation.thermal_liquid.thermal_liquid\"},{\"id\":\"C\",\"label\":\"C\",\"type\":\"foundation.mechanical.translational.translational\"},{\"id\":\"H\",\"label\":\"H\",\"type\":\"foundation.thermal.thermal\"}],\"Right\":[{\"id\":\"R\",\"label\":\"R\",\"type\":\"foundation.mechanical.translational.translational\"}],\"Top\":[]}"
  Expansion Tank Inlet : fl_lib/Thermal Liquid/Elements/Local Restriction (TL)  restriction_type=foundation.enum.restriction_type.fixed  restriction_area=pi*10^2 mm^2  min_area=1e-10 m^2  max_area=0.005 m^2  area=pi*11^2 mm^2  Cd=0.7  pressure_recovery=0  Re_c=12
      settings: SourceProductBaseCode=PW,SS,VE
  Insulator Expansion Tank : fl_lib/Thermal/Thermal Elements/Perfect Insulator  T_specify=off  T_priority=High  T=0 K  T_nominal_specify=off  T_nominal_unit=K  T_nominal_value=1
      settings: SourceProductBaseCode=PW,SS,VE
  MTRef : fl_lib/Mechanical/Translational Elements/Mechanical Translational Reference
      settings: SourceProductBaseCode=PW,SS,VE
  MTRef Air Stiffness : fl_lib/Mechanical/Translational Elements/Mechanical Translational Reference
      settings: SourceProductBaseCode=PW,SS,VE
  A : PMIOPort  Side=Left
  connections:
  MTRef/LConn1 -- Expansion Tank/LConn2
  Insulator Expansion Tank/LConn1 -- Expansion Tank/LConn3
  Expansion Tank Inlet/LConn1 -- A/RConn1
  Expansion Tank Inlet/RConn1 -- Expansion Tank/LConn1
  Air Stiffness/LConn1 -- Expansion Tank/RConn1
  Air Stiffness/RConn1 -- MTRef Air Stiffness/LConn1

== system ssc_auto_ev_20b/Step 2: Multirate Model/Cooling System/Heat Exchanger Characteristic ==
  Characteristic : Subsystem
  Heat Flow Source : fl_lib/Thermal/Thermal Sources/Controlled Heat Flow Rate Source
      settings: SourceProductBaseCode=PW,SS,VE
  Mass Flow Rate & Thermal Flux Sensor (TL) : fl_lib/Thermal Liquid/Sensors/Mass & Energy Flow Rate Sensor (TL)
      settings: SourceProductBaseCode=PW,SS,VE  InternalSimscapePortConfiguration="{\"Bottom\":[],\"Left\":[{\"id\":\"A\",\"label\":\"A\",\"type\":\"foundation.thermal_liquid.thermal_liquid\"}],\"Right\":[{\"id\":\"B\",\"label\":\"B\",\"type\":\"foundation.thermal_liquid.thermal_liquid\"},{\"id\":\"M\",\"label\":\"M\",\"type\":\"output\"},{\"id\":\"PHI\",\"label\":\"Phi\",\"type\":\"output\"}],\"Top\":[]}"
  Temperature Sensor : fl_lib/Thermal/Thermal Sensors/Temperature Sensor
      settings: SourceProductBaseCode=PW,SS,VE
  ThRef : fl_lib/Thermal/Thermal Elements/Thermal Reference
      settings: SourceProductBaseCode=PW,SS,VE
  HMotor : PMIOPort  Side=Right
  B : PMIOPort  Port=2  Side=Right
  Hp : PMIOPort  Port=3  Side=Left
  A : PMIOPort  Port=4  Side=Left
  TIn : PMIOPort  Port=5  Side=Left
  connections:
  Characteristic/RConn1 -- Heat Flow Source/RConn1
  Characteristic/LConn2 -- TIn/RConn1
  Mass Flow Rate & Thermal Flux Sensor (TL)/RConn2 -- Characteristic/LConn1
  Temperature Sensor/RConn2 -- Characteristic/LConn3
  A/RConn1 -- Mass Flow Rate & Thermal Flux Sensor (TL)/LConn1
  Heat Flow Source/LConn1 -- Hp/RConn1
  ThRef/LConn1 -- Temperature Sensor/RConn1
  HMotor/RConn1 -- Temperature Sensor/LConn1 -- Heat Flow Source/RConn2
  Mass Flow Rate & Thermal Flux Sensor (TL)/RConn1 -- B/RConn1

== system ssc_auto_ev_20b/Step 2: Multirate Model/Cooling System/Sensing Inlet Temperature ==
  Pressure & Temperature Sensor (TL) : fl_lib/Thermal Liquid/Sensors/Pressure & Temperature Sensor (TL)
      settings: SourceProductBaseCode=PW,SS,VE  InternalSimscapePortConfiguration="{\"Bottom\":[],\"Left\":[{\"id\":\"A\",\"label\":\"A\",\"type\":\"foundation.thermal_liquid.thermal_liquid\"}],\"Right\":[{\"id\":\"B\",\"label\":\"B\",\"type\":\"foundation.thermal_liquid.thermal_liquid\"},{\"id\":\"P\",\"label\":\"P\",\"type\":\"output\"},{\"id\":\"T\",\"label\":\"T\",\"type\":\"output\"}],\"Top\":[]}"
  TLRef : fl_lib/Thermal Liquid/Elements/Absolute Reference (TL)
      settings: SourceProductBaseCode=PW,SS,VE
  A : PMIOPort  Side=Left
  T : PMIOPort  Port=2  Side=Right
  connections:
  TLRef/LConn1 -- Pressure & Temperature Sensor (TL)/RConn1
  Pressure & Temperature Sensor (TL)/LConn1 -- A/RConn1
  Pressure & Temperature Sensor (TL)/RConn3 -- T/RConn1

== system ssc_auto_ev_20b/Step 2: Multirate Model/Cooling System/Sensing Temperature ==
  Pressure & Temperature Sensor (TL) : fl_lib/Thermal Liquid/Sensors/Pressure & Temperature Sensor (TL)
      settings: SourceProductBaseCode=PW,SS,VE  InternalSimscapePortConfiguration="{\"Bottom\":[],\"Left\":[{\"id\":\"A\",\"label\":\"A\",\"type\":\"foundation.thermal_liquid.thermal_liquid\"}],\"Right\":[{\"id\":\"B\",\"label\":\"B\",\"type\":\"foundation.thermal_liquid.thermal_liquid\"},{\"id\":\"P\",\"label\":\"P\",\"type\":\"output\"},{\"id\":\"T\",\"label\":\"T\",\"type\":\"output\"}],\"Top\":[]}"
  TLRef : fl_lib/Thermal Liquid/Elements/Absolute Reference (TL)
      settings: SourceProductBaseCode=PW,SS,VE
  T : PMIOPort  Side=Right
  A : PMIOPort  Port=2  Side=Left
  connections:
  A/RConn1 -- Pressure & Temperature Sensor (TL)/LConn1
  TLRef/LConn1 -- Pressure & Temperature Sensor (TL)/RConn1
  Pressure & Temperature Sensor (TL)/RConn3 -- T/RConn1

== system ssc_auto_ev_20b/Step 2: Multirate Model/Driver and Environment/Bus ==
  In : Inport
  Wi : Inport  Port=2
  Br : Inport  Port=3
  Bus Creator : BusCreator  Inputs=3
  b : Outport  VectorParamsAs1DForOutWhenUnconnected=off
  wires:
  In/1 -> Bus Creator/1  "Incline"
  Br/1 -> Bus Creator/3  "Brake pedal"
  Bus Creator/1 -> b/1
  Wi/1 -> Bus Creator/2  "Wind speed"

== system ssc_auto_ev_20b/Step 2: Multirate Model/Driver and Environment/Inclinometer ==
  a : Inport
  Trigonometric Function : Trigonometry
  d2r : Gain  Gain=pi/180
  g : Gain  Gain=gravity
  y : Outport  VectorParamsAs1DForOutWhenUnconnected=off
  wires:
  g/1 -> y/1
  d2r/1 -> Trigonometric Function/1
  a/1 -> d2r/1
  Trigonometric Function/1 -> g/1

== system ssc_auto_ev_20b/Step 2: Multirate Model/Motor Drive/DC Motor1 ==
  Inertia : fl_lib/Mechanical/Rotational Elements/Inertia  inertia=0.01 kg*m^2  num_ports=foundation.enum.numPorts2.one  w_specify=off  w_priority=High  w=0 rad/s  w_nominal_specify=off  w_nominal_unit=rad/s  w_nominal_value=1  t_specify=off  t_priority=High  t=0 N*m  t_nominal_specify=off  t_nominal_unit=N*m  t_nominal_value=1
      settings: SourceProductBaseCode=PW,SS,VE
  Rotational Electromechanical Converter : fl_lib/Electrical/Electrical Elements/Rotational Electromechanical Converter  K=1 N*m/A  i_specify=off  i_priority=High  i=0 A  i_nominal_specify=off  i_nominal_unit=A  i_nominal_value=1  v_specify=off  v_priority=High  v=0 V  v_nominal_specify=off  v_nominal_unit=V  v_nominal_value=1  t_specify=off  t_priority=High  t=0 N*m  t_nominal_specify=off  t_nominal_unit=N*m  t_nominal_value=1  w_specify=off  w_priority=High  w=0 rad/s  w_nominal_specify=off  w_nominal_unit=rad/s  w_nominal_value=1
      settings: SourceProductBaseCode=PW,SS,VE
  Thermal Resistor : fl_lib/Electrical/Electrical Elements/Thermal Resistor  R0=1 Ohm  T0=298.15 K  alpha=50e-6 1/K  tc=30 s  K_d=100 W/K  T_specify=off  T_priority=High  T=300 K  T_nominal_specify=off  T_nominal_unit=K  T_nominal_value=1
      settings: SourceProductBaseCode=PW,SS,VE  InternalSimscapePortConfiguration="{\"Bottom\":[],\"Left\":[{\"id\":\"H\",\"label\":\"H\",\"type\":\"foundation.thermal.thermal\"},{\"id\":\"p\",\"label\":\"+\",\"type\":\"foundation.electrical.electrical\"}],\"Right\":[{\"id\":\"n\",\"label\":\"-\",\"type\":\"foundation.electrical.electrical\"}],\"Top\":[]}"
  V+ : PMIOPort  Side=Left
  R : PMIOPort  Port=2  Side=Right
  C : PMIOPort  Port=3  Side=Right
  V- : PMIOPort  Port=4  Side=Left
  H : PMIOPort  Port=5  Side=Left
  connections:
  V-/RConn1 -- Rotational Electromechanical Converter/RConn1
  Thermal Resistor/LConn2 -- V+/RConn1
  Rotational Electromechanical Converter/LConn1 -- Thermal Resistor/RConn1
  Rotational Electromechanical Converter/LConn2 -- Inertia/LConn1 -- R/RConn1
  Rotational Electromechanical Converter/RConn2 -- C/RConn1
  H/RConn1 -- Thermal Resistor/LConn1
